simulink model "DPT_Update"  (R2023b)
settings: Solver=VariableStepAuto  StartTime=0.0  StopTime=0.0003  RelTol=1e-3
values from neighbouring files (symbols this model uses):
  Cb = (Lload*Itest^2)/(2*Vdc*deltaVdc-deltaVdc^2)    (= 8.27194361832e-05)    [DPT.m]
  Lload = 464.6*10^-6    (= 0.0004646)    [DPT.m]
  T1 = Lload*Itest/Vdc    (= 2.76547619048e-05)    [DPT.m]
  T2 = 5 * 10^-6    (= 5e-06)    [DPT.m]
  T3 = 5 * 10^-6    (= 5e-06)    [DPT.m]
  Tini = 0.0001    [DPT.m]
  Vdc = 420    [DPT.m]
libraries: spsMosfetLib x4, spsSeriesRLCBranchLib x2, spsCurrentMeasurementLib x1, spsVoltageMeasurementLib x1, spsDCVoltageSourceLib x1, sps_lib x1
settings Model: PacingRate=10  Creator=carlo  LastModifiedBy=carlo

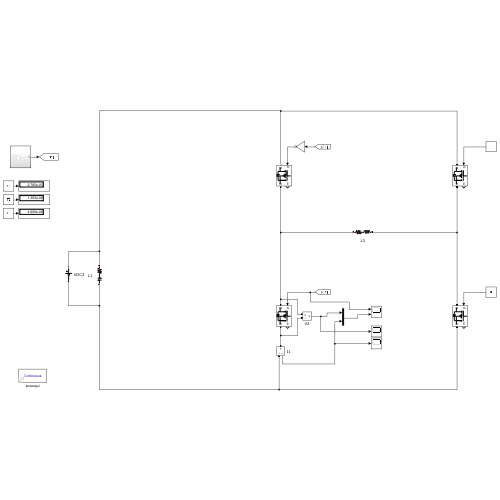
[thumbnail: Simulink's stored preview of the top-level diagram]
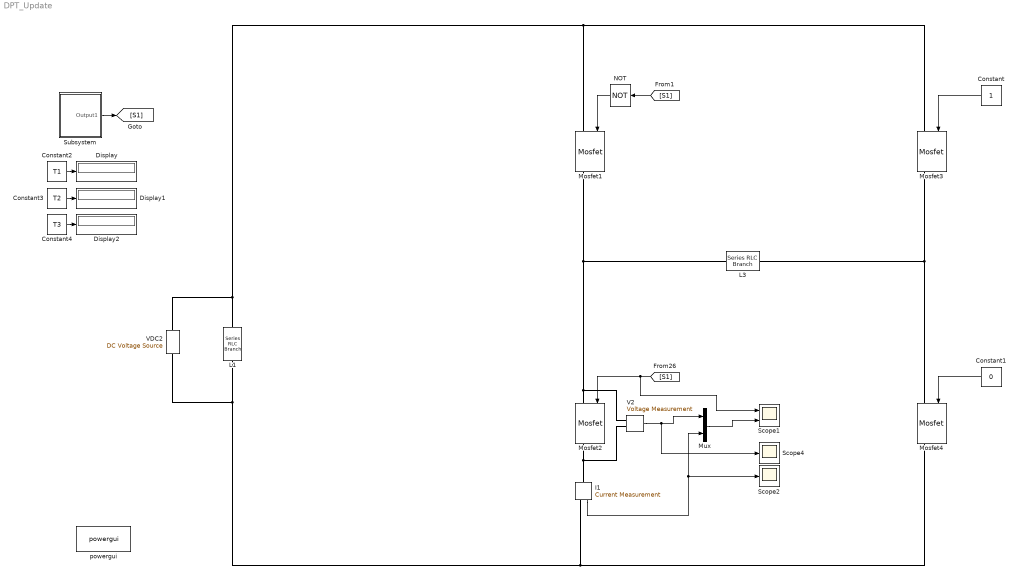
== system DPT_Update ==
  Constant : Constant
  Constant1 : Constant  Value=0
  Constant2 : Constant  Value=T1
  Constant3 : Constant  Value=T2
  Constant4 : Constant  Value=T3
  Display : Display
  Display1 : Display
  Display2 : Display
  I1 : spsCurrentMeasurementLib/Current Measurement  PhasorSimulation=off  OutputType=Complex  PSBequivalent=0
  L1 : spsSeriesRLCBranchLib/Series RLC Branch  LConnTagsString=__new0  RConnTagsString=__new0  BranchType=RC  Resistance=0.01  Inductance=Lload  SetiL0=off  InitialCurrent=0  Capacitance=Cb  Setx0=on  InitialVoltage=420  Measurements=None
  L3 : spsSeriesRLCBranchLib/Series RLC Branch  LConnTagsString=__new0  RConnTagsString=__new0  BranchType=RL  Resistance=0  Inductance=Lload  SetiL0=off  InitialCurrent=0  Capacitance=1e-6  Setx0=off  InitialVoltage=0  Measurements=None
  Mosfet{1..4} (4 alike) : spsMosfetLib/Mosfet  Ron=0.013  Lon=0  Rd=0.05689  Vfd=3.3  IC=0  Rs=1e5  Cs=inf  Measurements=on
  Mux : Mux  Inputs=2
  NOT : Logic  Operator=NOT  IconShape=distinctive  AllPortsSameDT=off  OutDataTypeStr=boolean
  Scope1 : Scope  NumInputPorts=2
  Scope2 : Scope
  Scope4 : Scope
  Subsystem : Subsystem
  V2 : spsVoltageMeasurementLib/Voltage Measurement  PhasorSimulation=off  OutputType=Complex  PSBequivalent=0
  VDC2 : spsDCVoltageSourceLib/DC Voltage Source  Amplitude=Vdc  Measurements=None
  powergui : sps_lib/powergui  Priority=1  SimulationMode=Continuous  SampleTime=50e-6  frequency=60  Iterations=50  frequencyindice=0  Pbase=100e6  ErrMax=1e-4  UnitsV=kV  UnitsW=MW  buscounter=0  FunctionMessages=off  echomessages=off  EnableUseOfTLC=off  CurrentSourceSwitches=off  DisableSnubberDevices=off  DisableRonSwitches=off  DisableVfSwitches=off  DisplayEquations=off  AutomaticDiscreteSolvers=off  SolverType=Tustin/Backward Euler (TBE)  Interpol=off  ExternalGateDelay=off  methode=off  Ts=100  x0status=blocks  SPID=on  SwTol=0  HookPort=off  NonlinearTolerance=1e-4  nMaxIteration=100  ContinueOnMaxIteration=off  RestoreLinks=warning  ResistiveCurrentMeasurement=off  Frange=[0:2:500]  Ylog=off  Xlog=on  ShowGrid=off  save=off  variable=ZData  structure=0  ZoomFFT=off  StartTime=0.0  cycles=1  DisplayStyle=1  fundamental=60  FreqAxis=off  MaxFrequency=1000  frequencyindicesteady=1  RmsSteady=1  display=off
  wires:
  [S1] -> Scope1/1, Mosfet2/1
  Subsystem/1(Output1) -> [S1]
  [S1] -> NOT/1
  NOT/1 -> Mosfet1/1
  Constant1/1 -> Mosfet4/1
  Constant/1 -> Mosfet3/1
  I1/1 -> Scope2/1, Mux/2
  V2/1 -> Scope4/1, Mux/1
  Mux/1 -> Scope1/2
  Constant2/1 -> Display/1
  Constant3/1 -> Display1/1
  Constant4/1 -> Display2/1
  connections:
  Mosfet2/LConn1 -- V2/LConn1 -- L3/LConn1 -- Mosfet1/RConn1
  Mosfet4/LConn1 -- L3/RConn1 -- Mosfet3/RConn1
  VDC2/RConn1 -- Mosfet3/LConn1 -- Mosfet1/LConn1 -- L1/LConn1
  VDC2/LConn1 -- I1/RConn1 -- Mosfet4/RConn1 -- L1/RConn1
  Mosfet2/RConn1 -- V2/LConn2 -- I1/LConn1

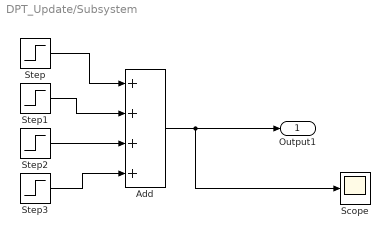
== system DPT_Update/Subsystem ==
  Add : Sum  Inputs=++++
  Scope : Scope
  Step : Step  Time=Tini  SampleTime=0
  Step1 : Step  Time=Tini + T1  After=-1  SampleTime=0
  Step2 : Step  Time=Tini + T1+ T2  SampleTime=0
  Step3 : Step  Time=Tini + T1 + T2 + T3  After=-1  SampleTime=0
  Output1 : Outport
  wires:
  Step2/1 -> Add/3
  Add/1 -> Output1/1, Scope/1
  Step3/1 -> Add/4
  Step/1 -> Add/1
  Step1/1 -> Add/2
